simulink model "Temporal_logic"  (R2020a)
settings: Solver=VariableStepAuto  StartTime=0.0  StopTime=10.0  RelTol=1e-3
settings Model: Creator=apple  LastModifiedBy=apple

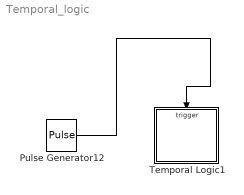
== system Temporal_logic ==
  Pulse Generator12 : DiscretePulseGenerator  PulseType=Time based  Period=1  PulseWidth=50
  Temporal Logic1 : Stateflow chart  TreatAsAtomicUnit=on
  wires:
  Pulse Generator12/1 -> Temporal Logic1/Trigger

== stateflow chart Temporal_logic/Temporal Logic1 ==
  state A
    du: x = 2;
    ex:x = 1;
    on at(2,E): x = x-3;
    on every(1,E): x = x+1;
    state A1
      ex:x = temporalCount(E);
    (default) -> A1
    (junction 27) -> A1
    A1 -> (junction 27)
  state B
    en: x=x+1;
  (default) -> A : {x=0;}
  A -> B : after(3,E)/{x = temporalCount(E);}
  B -> A
  data: x local
  events: E input EITHER_EDGE_EVENT
